simulink model "sim3"  (R2023b)
settings: Solver=VariableStepAuto  StartTime=0.0  StopTime=100  RelTol=1e-3
settings Model: Creator=anura  LastModifiedBy=anura

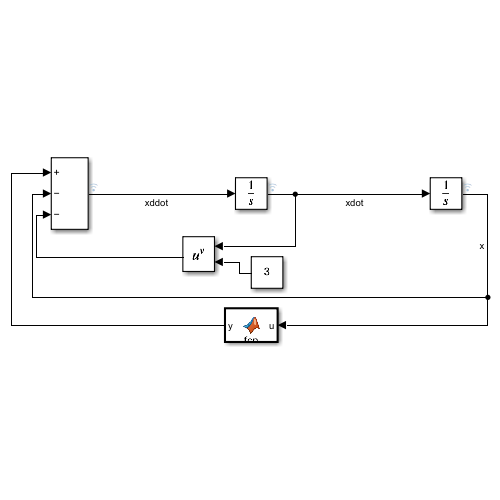
[thumbnail: Simulink's stored preview of the top-level diagram]
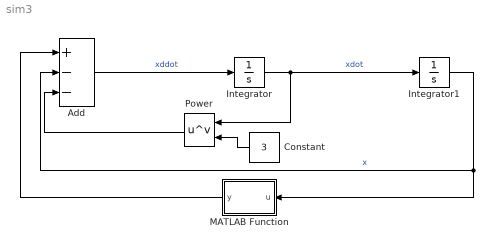
== system sim3 ==
  Add : Sum  Inputs=+--
  Constant : Constant  Value=3
  Integrator : Integrator  InitialCondition=-0.2
  Integrator1 : Integrator  InitialCondition=2
  MATLAB Function : MATLAB Function  TreatAsAtomicUnit=on
  Power : Math  Operator=pow
  wires:
  Integrator/1 -> Integrator1/1, Power/1  "xdot"
  Add/1 -> Integrator/1  "xddot"
  Constant/1 -> Power/2
  Power/1 -> Add/3
  MATLAB Function/1(y) -> Add/1
  Integrator1/1 -> MATLAB Function/1(u), Add/2  "x"

== matlab function sim3/MATLAB Function ==
  data: u input; y output
function y = fcn(u)

y = sin(u)^2;

end
